simulink model "nominal_model"  (R2023b)
settings: Solver=VariableStepAuto  StartTime=0.0  StopTime=inf  FixedStep=0.1  RelTol=1e-3
undefined symbols (not defined in the file): DiscIntNeverNeededParam
libraries: simulink x2
settings Model: Creator=awcm9  LastModifiedBy=awcm9

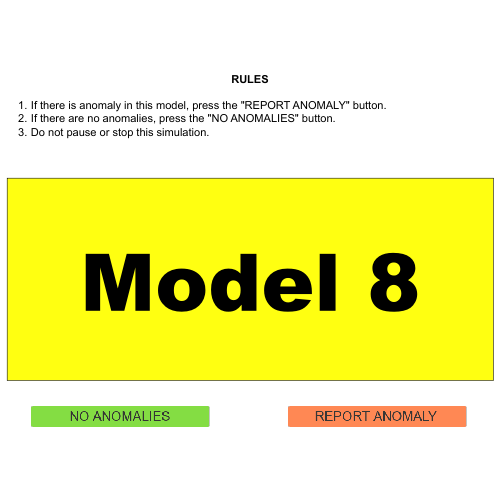
[thumbnail: Simulink's stored preview of the top-level diagram]
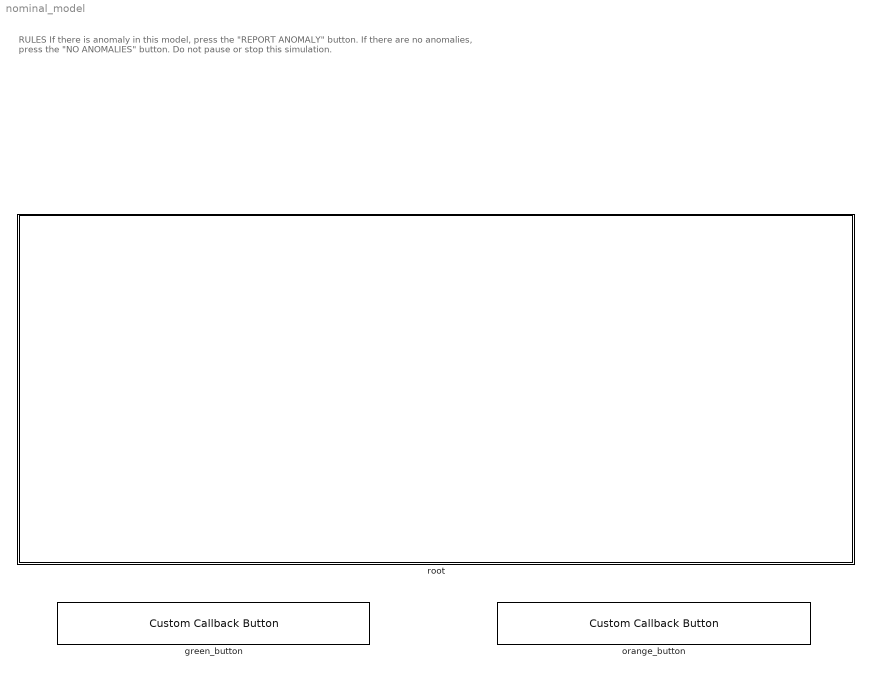
== system nominal_model ==
  note: RULES
      |
      | If there is anomaly in this model, press the "REPORT ANOMALY" button.
      | If there are no anomalies, press the "NO ANOMALIES" button.
      | Do not pause or stop this simulation.
  green_button : CustomCallbackButton  Configuration="{\"components\":[{\"name\":\"BackgroundImageComponent\",\"settings\":{\"image\":{\"size\":[0,0],\"src\":\"default\",\"srcOrientation\":\"Right\"},\"position\":[0,0,1,1]}},{\"name\":\"ButtonStateComponent\",\"settings\":{\"buttonType\":\"momentary\",\"clickFcn\":\"set_param(gcbh, \\\"UserData\\\", true);\\nset_param(gcs, \\\"SimulationCommand\\\", \\\"Stop\\\");\",\"onValue\":1,\"position\":[0,0,1,1],\"pressDelay\":\"500\",\"pressFcn\":\"\",\"repeatInterval\":\"0\",\"states\":[{\"horizontalAlignment\":\"center\",\"image\":{\"position\":[0,0,1,1],\"size\":[1,1],\"src\":\"default\",\"srcOrientation\":\"Right\"},\"label\":{\"color\":[0,0,0],\"icon\":{\"size\":[0,0],\"src\":\"default\",\"srcOrientation\":\"Right\"},\"iconPlacement\":\"left\",\"opacity\":1,\"show\":true,\"text\":{\"content\":\"NO ANOMALIES\",\"font\":\"Helvetica\",\"fontSize\":19.200000000000003}},\"labelOffset\":[0,0],\"verticalAlignment\":\"middle\"},{\"horizontalAlignment\":\"center\",\"image\":{\"position\":[0,0,1,1],\"size\":[1,1],\"src\":\"default\",\"srcOrientation\":\"Right\"},\"label\":{\"color\":[0,0,0],\"icon\":{\"size\":[0,0],\"src\":\"default\",\"srcOrientation\":\"Right\"},\"iconPlacement\":\"left\",\"opacity\":1,\"show\":true,\"text\":{\"content\":\"NO ANOMALIES\",\"font\":\"Helvetica\",\"fontSize\":19.200000000000003}},\"labelOffset\":[0,0],\"verticalAlignment\":\"middle\"},{\"horizontalAlignment\":\"center\",\"image\":{\"position\":[0,0,1,1],\"size\":[1,1],\"src\":\"default\",\"srcOrientation\":\"Right\"},\"label\":{\"color\":[0,0,0],\"icon\":{\"size\":[0,0],\"src\":\"default\",\"srcOrientation\":\"Right\"},\"iconPlacement\":\"left\",\"opacity\":1,\"show\":true,\"text\":{\"content\":\"NO ANOMALIES\",\"font\":\"Helvetica\",\"fontSize\":19.200000000000003}},\"labelOffset\":[0,0],\"verticalAlignment\":\"middle\"},{\"horizontalAlignment\":\"center\",\"image\":{\"position\":[0,0,1,1],\"size\":[1,1],\"src\":\"default\",\"srcOrientation\":\"Right\"},\"label\":{\"color\":[0,0,0],\"icon\":{\"size\":[0,0],\"src\":\"default\",\"srcOrientation\":\"Right\"},\"iconPlacement\":\"left\",\"opacity\":1,\"show\":true,\"text\":{\"content\":\"NO ANOMALIES\",\"font\":\"Helvetica\",\"fontSize\":19.200000000000003}},\"labelOffset\":[0,0],\"verticalAlignment\":\"middle\"}]}},{\"name\":\"ForegroundImageComponent\",\"settings\":{\"image\":{\"size\":[0,0],\"src\":\"default\",\"srcOrientation\":\"Right\"},\"isForeground\":1,\"position\":[0,0,1,1]}}],\"settings\":{\"BindingType\":\"standalone\",\"backgroundColor\":[244,244,244,1],\"backgroundOffset\":0.2,\"backgroundOpacity\":1,\"fixedAspectRatio\":\"off\",\"foregroundColor\":[0.01176470588,0.01176470588,0.01176470588,1],\"migratedFromLegacy\":true,\"useBackgroundColor\":true,\"variant\":\"callback\",\"version\":\"R2023a\"},\"type\":\"Button\"}"  CustomBackgroundColor="{\"color\":[0.39215686274509803,0.8313725490196079,0.07450980392156863],\"show\":true}"
  orange_button : CustomCallbackButton  Configuration="{\"components\":[{\"name\":\"BackgroundImageComponent\",\"settings\":{\"image\":{\"size\":[0,0],\"src\":\"default\",\"srcOrientation\":\"Right\"},\"position\":[0,0,1,1]}},{\"name\":\"ButtonStateComponent\",\"settings\":{\"buttonType\":\"momentary\",\"clickFcn\":\"set_param(gcbh, \\\"UserData\\\", true);\\nset_param(gcs, \\\"SimulationCommand\\\", \\\"Stop\\\");\",\"onValue\":1,\"position\":[0,0,1,1],\"pressDelay\":\"500\",\"pressFcn\":\"\",\"repeatInterval\":\"0\",\"states\":[{\"horizontalAlignment\":\"center\",\"image\":{\"position\":[0,0,1,1],\"size\":[1,1],\"src\":\"default\",\"srcOrientation\":\"Right\"},\"label\":{\"color\":[0.01176470588,0.01176470588,0.01176470588,1],\"icon\":{\"size\":[0,0],\"src\":\"default\",\"srcOrientation\":\"Right\"},\"iconPlacement\":\"left\",\"opacity\":1,\"show\":true,\"text\":{\"content\":\"REPORT ANOMALY\",\"font\":\"Arial\",\"fontSize\":19.200000000000003}},\"labelOffset\":[0,0],\"verticalAlignment\":\"middle\"},{\"horizontalAlignment\":\"center\",\"image\":{\"position\":[0,0,1,1],\"size\":[1,1],\"src\":\"default\",\"srcOrientation\":\"Right\"},\"label\":{\"color\":[0.01176470588,0.01176470588,0.01176470588,1],\"icon\":{\"size\":[0,0],\"src\":\"default\",\"srcOrientation\":\"Right\"},\"iconPlacement\":\"left\",\"opacity\":1,\"show\":true,\"text\":{\"content\":\"REPORT ANOMALY\",\"font\":\"Arial\",\"fontSize\":19.200000000000003}},\"labelOffset\":[0,0],\"verticalAlignment\":\"middle\"},{\"horizontalAlignment\":\"center\",\"image\":{\"position\":[0,0,1,1],\"size\":[1,1],\"src\":\"default\",\"srcOrientation\":\"Right\"},\"label\":{\"color\":[0.01176470588,0.01176470588,0.01176470588,1],\"icon\":{\"size\":[0,0],\"src\":\"default\",\"srcOrientation\":\"Right\"},\"iconPlacement\":\"left\",\"opacity\":1,\"show\":true,\"text\":{\"content\":\"REPORT ANOMALY\",\"font\":\"Arial\",\"fontSize\":19.200000000000003}},\"labelOffset\":[0,0],\"verticalAlignment\":\"middle\"},{\"horizontalAlignment\":\"center\",\"image\":{\"position\":[0,0,1,1],\"size\":[1,1],\"src\":\"default\",\"srcOrientation\":\"Right\"},\"label\":{\"color\":[0.01176470588,0.01176470588,0.01176470588,1],\"icon\":{\"size\":[0,0],\"src\":\"default\",\"srcOrientation\":\"Right\"},\"iconPlacement\":\"left\",\"opacity\":1,\"show\":true,\"text\":{\"content\":\"REPORT ANOMALY\",\"font\":\"Arial\",\"fontSize\":19.200000000000003}},\"labelOffset\":[0,0],\"verticalAlignment\":\"middle\"}]}},{\"name\":\"ForegroundImageComponent\",\"settings\":{\"image\":{\"size\":[0,0],\"src\":\"default\",\"srcOrientation\":\"Right\"},\"isForeground\":1,\"position\":[0,0,1,1]}}],\"settings\":{\"BindingType\":\"standalone\",\"backgroundColor\":[244,244,244,1],\"backgroundOffset\":0.2,\"backgroundOpacity\":1,\"fixedAspectRatio\":\"off\",\"foregroundColor\":[0.01176470588,0.01176470588,0.01176470588,1],\"migratedFromLegacy\":true,\"useBackgroundColor\":true,\"variant\":\"callback\",\"version\":\"R2023a\"},\"type\":\"Button\"}"  CustomBackgroundColor="{\"color\":[1,0.411765,0.160784],\"show\":true}"
  root : Subsystem
      mask Display: disp('Model 8');

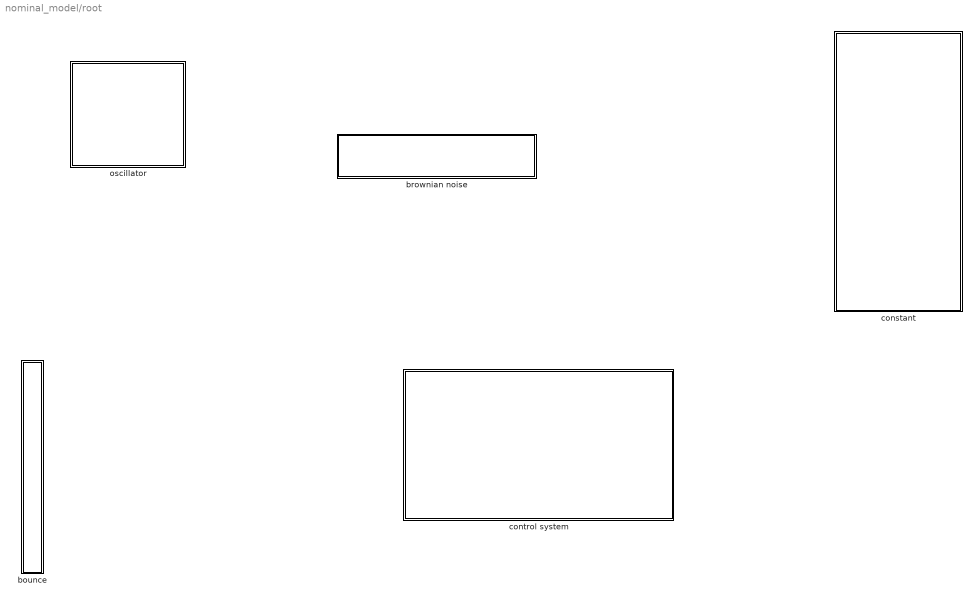
== system nominal_model/root ==
  bounce : Subsystem
  brownian noise : Subsystem
  constant : Subsystem
  control system : Subsystem
  oscillator : Subsystem

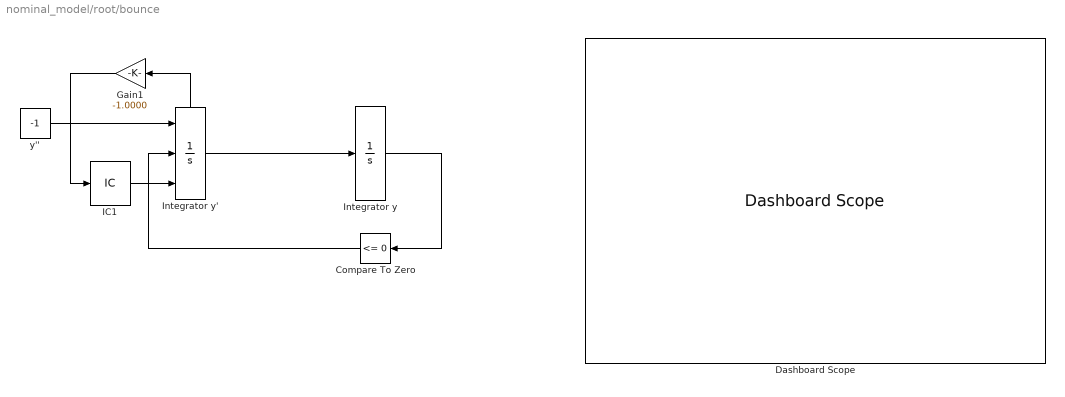
== system nominal_model/root/bounce ==
  Compare To Zero : simulink/Logic and Bit Operations/Compare To Zero  relop=<=  OutDataTypeStr=boolean
  Dashboard Scope : DashboardScope  ShowInitialText=off  TimeSpan=10  Ymin=-.25  Ymax=1.25  ScaleAtStop=off  UpdateMode=Scroll
  Gain1 : Gain  Gain=-1.0000
  IC1 : InitialCondition
  Integrator y : Integrator  InitialCondition=0.5  LimitOutput=on  UpperSaturationLimit=10  LowerSaturationLimit=0  ZeroCross=off
  Integrator y' : Integrator  ExternalReset=rising  InitialConditionSource=external  ShowStatePort=on  ZeroCross=off
  y'' : Constant  Value=-1
  wires:
  Integrator y'/1 -> Integrator y/1
  y''/1 -> Integrator y'/1
  Gain1/1 -> IC1/1
  IC1/1 -> Integrator y'/3
  Integrator y'/State -> Gain1/1
  Compare To Zero/1 -> Integrator y'/2
  Integrator y/1 -> Compare To Zero/1

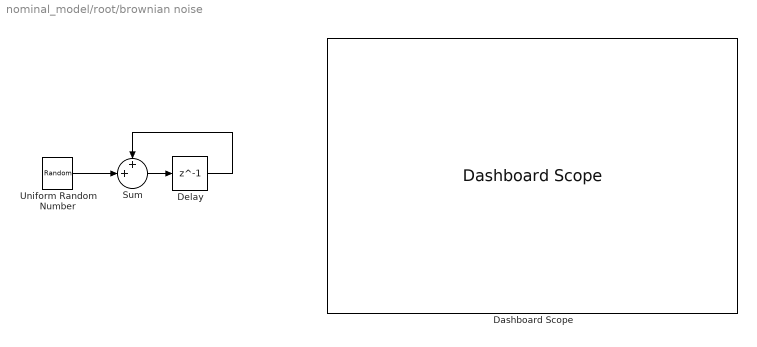
== system nominal_model/root/brownian noise ==
  Dashboard Scope : DashboardScope  ShowInitialText=off  TimeSpan=15  Ymin=-30  Ymax=30  ScaleAtStop=off
  Delay : Delay  DelayLength=1
  Sum : Sum  Inputs=++|
  Uniform Random Number : UniformRandomNumber  SampleTime=1
  wires:
  Uniform Random Number/1 -> Sum/2
  Delay/1 -> Sum/1
  Sum/1 -> Delay/1

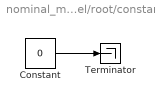
== system nominal_model/root/constant ==
  Constant : Constant  Value=0  SampleTime=1
  Terminator : Terminator
  wires:
  Constant/1 -> Terminator/1

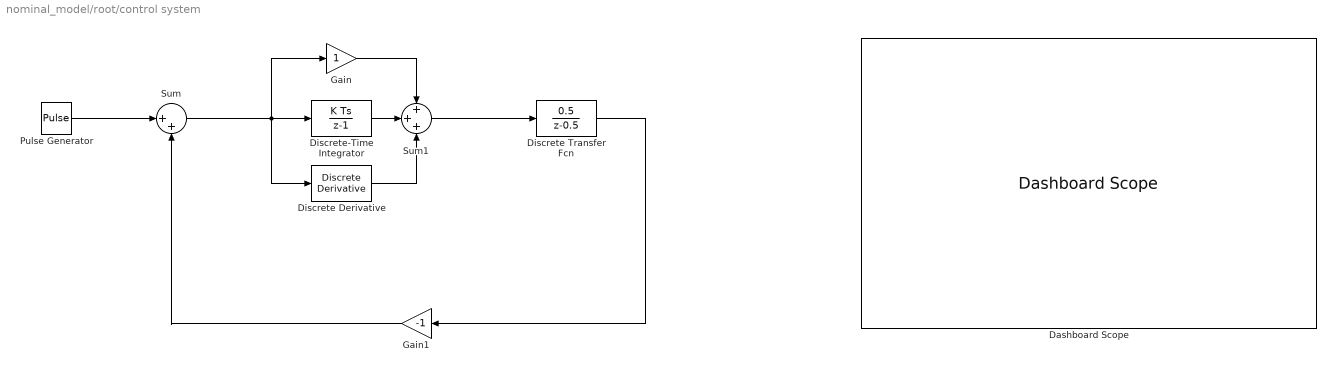
== system nominal_model/root/control system ==
  Dashboard Scope : DashboardScope  ShowInitialText=off  TimeSpan=20  Ymin=-1.0  Ymax=2.0  ScaleAtStop=off
  Discrete Transfer Fcn : DiscreteTransferFcn  Numerator=[0.5]  Denominator=[1 -0.5]
  Discrete Derivative : simulink/Discrete/Discrete Derivative  gainval=0.1  ICPrevScaledInput=0.0  OutMin=[]  OutMax=[]  OutDataType=fixdt(1, 16)  OutScaling=2^-10  DoSatur=off
  Discrete-Time Integrator : DiscreteIntegrator  gainval=0.75  SampleTime=-1  ICPrevOutput=DiscIntNeverNeededParam  ICPrevScaledInput=DiscIntNeverNeededParam
  Gain : Gain
  Gain1 : Gain  Gain=-1
  Pulse Generator : DiscretePulseGenerator  Period=20  PulseWidth=10
  Sum : Sum  Inputs=|++
  Sum1 : Sum  Inputs=+++
  wires:
  Pulse Generator/1 -> Sum/1
  Sum/1 -> Gain/1, Discrete Derivative/1, Discrete-Time Integrator/1
  Discrete Transfer Fcn/1 -> Gain1/1
  Gain/1 -> Sum1/1
  Sum1/1 -> Discrete Transfer Fcn/1
  Discrete-Time Integrator/1 -> Sum1/2
  Discrete Derivative/1 -> Sum1/3
  Gain1/1 -> Sum/2

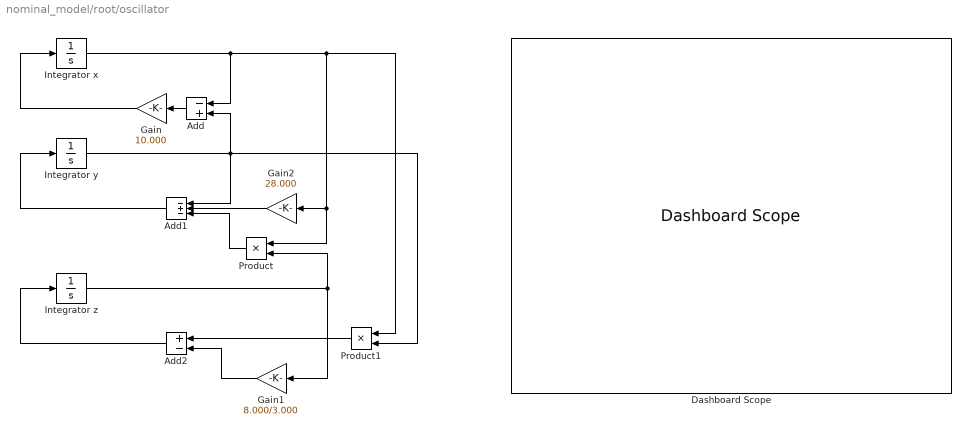
== system nominal_model/root/oscillator ==
  Add : Sum  Inputs=-+
  Add1 : Sum  Inputs=-+-
  Add2 : Sum  Inputs=+-
  Dashboard Scope : DashboardScope  ShowInitialText=off  TimeSpan=5  Ymin=-50  Ymax=50  ScaleAtStop=off
  Gain : Gain  Gain=10.000
  Gain1 : Gain  Gain=8.000/3.000
  Gain2 : Gain  Gain=28.000
  Integrator x : Integrator  InitialCondition=1
  Integrator y : Integrator
  Integrator z : Integrator
  Product : Product
  Product1 : Product
  wires:
  Integrator x/1 -> Add/1, Product1/1, Product/1, Gain2/1
  Integrator y/1 -> Product1/2, Add1/1, Add/2
  Add/1 -> Gain/1
  Integrator z/1 -> Gain1/1, Product/2
  Gain/1 -> Integrator x/1
  Gain2/1 -> Add1/2
  Product/1 -> Add1/3
  Add1/1 -> Integrator y/1
  Product1/1 -> Add2/1
  Gain1/1 -> Add2/2
  Add2/1 -> Integrator z/1
